simulink model "PMSM_SMO"  (Simulink 10.0)
settings: Solver=ode45  StartTime=0.0  StopTime=0.1  RelTol=1e-3  EnableMultiTasking=on
libraries: powerlib x11, simulink x1
settings Model: Creator=jzxpc  LastModifiedBy=bhisma
settings DataIOCC: LimitDataPoints=on  SignalLoggingSaveFormat=ModelDataLogs
settings OptimizationCC: ExpressionDepthLimit=2147483647  InitFltsAndDblsToZero=on
settings DebuggingCC: SaveWithParameterizedLinksMsg=none  SignalResolutionControl=TryResolveAllWithWarning  FcnCallInpInsideContextMsg=warning  StateNameClashWarn=warning
settings SFSimCC: SimParseCustomCode=off
settings GRTTargetCC: TargetFcnLib=ansi_tfl_tmw.mat  GeneratePreprocessorConditionals=Disable all
settings ConfigComp: CovExternalEMLEnable=off

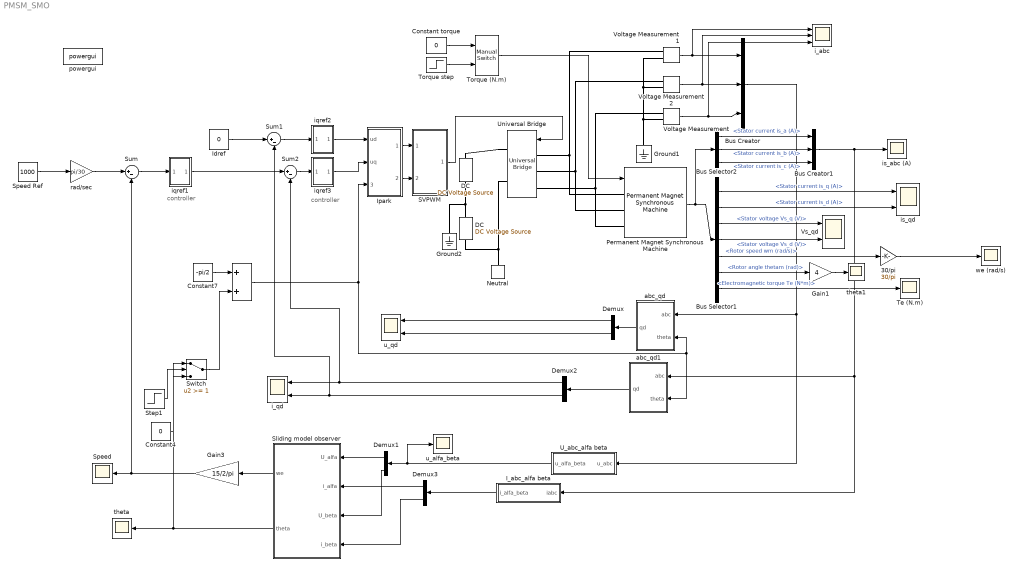
== system PMSM_SMO ==
  note: controller
  note: controller
  "  " : Sum
  30/pi : Gain  Gain=30/pi
  Bus Creator : BusCreator  Inputs=3
  Bus Creator1 : BusCreator  Inputs=3
  Bus Selector1 : BusSelector  OutputSignals=Stator current is_q (A),Stator current is_d (A),Stator voltage Vs_q (V),Stator voltage Vs_d (V),Rotor speed wm (rad/s),Rotor angle thetam (rad),Electromagnetic torque Te (N*m)
  Bus Selector2 : BusSelector  OutputSignals=Stator current is_a (A),Stator current is_b (A),Stator current is_c (A)
  Constant torque : Constant  Value=0
  Constant4 : Constant  Value=0
  Constant7 : Constant  Value=-pi/2
  DC : powerlib/Electrical Sources/DC Voltage Source  SystemSampleTime=-1  Amplitude=250  Measurements=None
      settings: SourceProductName=Simscape Electrical
  "DC " : powerlib/Electrical Sources/DC Voltage Source  SystemSampleTime=-1  Amplitude=250  Measurements=None
      settings: SourceProductName=Simscape Electrical
  Demux{,1..3} (4 alike) : Demux  Outputs=2
  Gain1 : Gain  Gain=4
  Gain3 : Gain  Gain=15/2/pi
  Ground1 : powerlib/Elements/Ground  PhysicalDomain=powersysdomain  SubClassName=unknown  LeftPortType=p1  RightPortType=p1  LConnTagsString=a
      settings: SourceProductName=Simscape Electrical
  Ground2 : powerlib/Elements/Ground  PhysicalDomain=powersysdomain  SubClassName=unknown  LeftPortType=p1  RightPortType=p1  LConnTagsString=a
      settings: SourceProductName=Simscape Electrical
  I_abc_alfa beta : Subsystem
  Idref : Constant  Value=0
  Ipark : Subsystem
  Neutral : powerlib/Elements/Neutral  PhysicalDomain=powersysdomain  SubClassName=unknown  LeftPortType=p1  RightPortType=p1  LConnTagsString=a  NodeNumber=10
      settings: SourceProductName=Simscape Electrical  SourceProductBaseCode=PS
  Permanent Magnet Synchronous Machine : powerlib/Machines/Permanent Magnet Synchronous Machine  SystemSampleTime=-1  FluxDistribution=Sinusoidal  MechanicalLoad=Torque Tm  PresetModel=No  ShowDetailedParameters=on  Resistance=1.9  Inductance=8.5e-3  dqInductances=[1e-2 1e-2]  MachineConstant=Flux linkage established by magnets (V.s)  Flux=0.353  VoltageCst=128.0542  TorqueCst=1.059  Flat=120  Mechanical=[7.24e-4 0.02e-6 2]  PolePairs=2  InitialConditions=[0,0, 0,0]  TsPowergui=0  TsBlock=-1
  SVPWM : Subsystem  TreatAsAtomicUnit=on
  Sliding model observer : Subsystem
  Speed : Scope
  Speed Ref : Constant  Value=1000
  Step1 : Step  Time=0.001  SampleTime=0
  Sum : Sum  Inputs=|+-
  Sum1 : Sum  Inputs=|+-
  Sum2 : Sum  Inputs=|+-
  Switch : Switch  Threshold=1
  Te (N.m) : Scope
  Torque (N.m) : simulink/Signal Routing/Manual Switch  SystemSampleTime=-1  sw=0  action=0  varsize=off
      settings: SourceProductName=Simulink  SourceProductBaseCode=SL
  Torque step : Step  Time=0  After=4  SampleTime=0
  U_abc_alfa beta : Subsystem
  Universal Bridge : powerlib/Power Electronics/Universal Bridge  SystemSampleTime=-1  Arms=3  SnubberResistance=1e5  SnubberCapacitance=inf  Device=IGBT / Diodes  Ron=1e-3  Lon=0  ForwardVoltages="[  0  0  ]"  ForwardVoltage=0  GTOparameters=[ 10e-6 , 20e-6 ]  IGBTparameters=[ 1e-6 , 2e-6 ]  Measurements=None  Measurements_2=None  converterType=Rectifier
      settings: SourceProductName=Simscape Electrical
  Voltage Measurement : powerlib/Measurements/Voltage Measurement  SystemSampleTime=-1  PhasorSimulation=off  OutputType=Complex  PSBequivalent=0
      settings: SourceProductName=Simscape Electrical
  Voltage Measurement1 : powerlib/Measurements/Voltage Measurement  SystemSampleTime=-1  PhasorSimulation=off  OutputType=Complex  PSBequivalent=0
      settings: SourceProductName=Simscape Electrical
  Voltage Measurement2 : powerlib/Measurements/Voltage Measurement  SystemSampleTime=-1  PhasorSimulation=off  OutputType=Complex  PSBequivalent=0
      settings: SourceProductName=Simscape Electrical
  Vs_qd : Scope  NumInputPorts=2
  abc_qd : Subsystem
  abc_qd1 : Subsystem
  i_abc : Scope  NumInputPorts=3
  "i_qd " : Scope  NumInputPorts=2
  iqref1 : Subsystem  mask(PI Controller){I=1.2, P=2, sat=[-50, 50]}
      mask prompts: I "Integral"; P "Proportional:"; sat "Minimum and maximum outputs:"
      mask init:
      | min=sat(1);max=sat(2);
      mask Display: disp('PI')
  iqref2 : Subsystem  mask(PI Controller){I=1000, P=10, sat=[-200, 200]}
      mask prompts: I "Integral"; P "Proportional:"; sat "Minimum and maximum outputs:"
      mask init:
      | min=sat(1);max=sat(2);
      mask Display: disp('PI')
  iqref3 : Subsystem  mask(PI Controller){I=1000, P=10, sat=[-200, 200]}
      mask prompts: I "Integral"; P "Proportional:"; sat "Minimum and maximum outputs:"
      mask init:
      | min=sat(1);max=sat(2);
      mask Display: disp('PI')
  is_abc (A) : Scope
  is_qd : Scope  NumInputPorts=2
  powergui : powerlib/powergui  SystemSampleTime=-1  SimulationMode=Continuous  SampleTime=50e-6  frequency=60  SPID=off  DisableSnubberDevices=off  DisableRonSwitches=off  DisableVfSwitches=off  SwTol=0  Interpol=off  frequencyindice=0  echomessages=off  HookPort=off  DisplayEquations=off  FunctionMessages=off  EnableUseOfTLC=off  x0status=blocks  RestoreLinks=warning  ResistiveCurrentMeasurement=off  Frange=[0:2:500]  Ylog=off  Xlog=on  ShowGrid=off  save=off  variable=ZData  ZoomFFT=on  StartTime=0.0  cycles=1  DisplayStyle=1  fundamental=60  FreqAxis=off  MaxFrequency=1000  frequencyindicesteady=1  RmsSteady=1  display=off  Ts=0  methode=off
      settings: SourceProductName=Simscape Electrical
  rad/sec : Gain  Gain=pi/30
  theta : Scope
  theta1 : Scope
  u_alfa_beta : Scope
  "u_qd " : Scope  NumInputPorts=2
  we (rad/s) : Scope
  wires:
  iqref2/1(Out_1) -> Ipark/1(ud)
  iqref3/1(Out_1) -> Ipark/2(uq)
  Ipark/1(ualpha) -> SVPWM/1(Ualfa)
  Ipark/2(ubeta) -> SVPWM/2(Ubeta)
  Sum/1 -> iqref1/1(In_1)
  Speed Ref/1 -> rad/sec/1
  Permanent Magnet Synchronous Machine/1 -> Bus Selector2/1, Bus Selector1/1
  Idref/1 -> Sum1/1
  Sum1/1 -> iqref2/1(In_1)
  Sum2/1 -> iqref3/1(In_1)
  iqref1/1(Out_1) -> Sum2/1
  Torque step/1 -> Torque (N.m)/2
  Constant torque/1 -> Torque (N.m)/1
  Voltage Measurement1/1 -> Bus Creator/1, i_abc/1
  Voltage Measurement2/1 -> Bus Creator/2, i_abc/2
  Voltage Measurement/1 -> Bus Creator/3, i_abc/3
  Bus Selector2/1 -> Bus Creator1/1  "<Stator current is_a (A)>"
  Bus Selector2/2 -> Bus Creator1/2  "<Stator current is_b (A)>"
  Bus Selector2/3 -> Bus Creator1/3  "<Stator current is_c (A)>"
  Bus Creator1/1 -> is_abc (A)/1, I_abc_alfa beta/1(iabc), abc_qd1/1(abc)
  Bus Selector1/1 -> is_qd/1  "<Stator current is_q (A)>"
  Bus Selector1/2 -> is_qd/2  "<Stator current is_d (A)>"
  Bus Selector1/3 -> Vs_qd/1  "<Stator voltage Vs_q (V)>"
  Bus Selector1/4 -> Vs_qd/2  "<Stator voltage Vs_d (V)>"
  Bus Selector1/5 -> 30/pi/1  "<Rotor speed wm (rad/s)>"
  Bus Selector1/6 -> Gain1/1  "<Rotor angle thetam (rad)>"
  Bus Selector1/7 -> Te (N.m)/1  "<Electromagnetic torque Te (N*m)>"
  30/pi/1 -> we (rad/s)/1
  Bus Creator/1 -> U_abc_alfa beta/1(u_abc), abc_qd/1(abc)
  Demux/1 -> "u_qd "/1
  Demux/2 -> "u_qd "/2
  abc_qd/1(qd) -> Demux/1
  Demux2/1 -> "i_qd "/1, Sum2/2
  Demux2/2 -> "i_qd "/2, Sum1/2
  abc_qd1/1(qd) -> Demux2/1
  U_abc_alfa beta/1(u_alfa_beta) -> Demux1/1, u_alfa_beta/1
  I_abc_alfa beta/1(i_alfa_beta) -> Demux3/1
  Demux1/1 -> Sliding model observer/1(U_alfa)
  Demux1/2 -> Sliding model observer/3(U_beta)
  Demux3/1 -> Sliding model observer/2(i_alfa)
  Demux3/2 -> Sliding model observer/4(i_beta)
  Gain3/1 -> Speed/1, Sum/2
  Sliding model observer/1(we) -> Gain3/1
  Sliding model observer/2(theta) -> Switch/1, theta/1
  Switch/1 -> "  "/2
  Step1/1 -> Switch/2
  Constant4/1 -> Switch/3
  Constant7/1 -> "  "/1
  "  "/1 -> Ipark/3(theta), abc_qd/2(theta), abc_qd1/2(theta)
  rad/sec/1 -> Sum/1
  SVPWM/1(Pulses) -> Universal Bridge/1
  Torque (N.m)/1 -> Permanent Magnet Synchronous Machine/1
  Gain1/1 -> theta1/1
  connections:
  Voltage Measurement1/LConn2 -- Voltage Measurement2/LConn2 -- Ground1/LConn1 -- Voltage Measurement/LConn2
  Universal Bridge/LConn1 -- Permanent Magnet Synchronous Machine/LConn1 -- Voltage Measurement1/LConn1
  Permanent Magnet Synchronous Machine/LConn2 -- Universal Bridge/LConn2 -- Voltage Measurement2/LConn1
  Universal Bridge/LConn3 -- Permanent Magnet Synchronous Machine/LConn3 -- Voltage Measurement/LConn1
  DC/RConn1 -- Ground2/LConn1 -- "DC "/LConn1
  DC/LConn1 -- Neutral/LConn1 -- Universal Bridge/RConn2
  Universal Bridge/RConn1 -- "DC "/RConn1

== system PMSM_SMO/I_abc_alfa beta ==
  iabc : Inport
  Fcn : Fcn  Expr=(2*u(1)-u(2)-u(3))/3
  Fcn1 : Fcn  Expr=(u(2)-u(3))/(3^(1/2))
  Mux2 : Mux  Inputs=2
  i_alfa_beta : Outport
  wires:
  Fcn1/1 -> Mux2/2
  Fcn/1 -> Mux2/1
  Mux2/1 -> i_alfa_beta/1
  iabc/1 -> Fcn1/1, Fcn/1

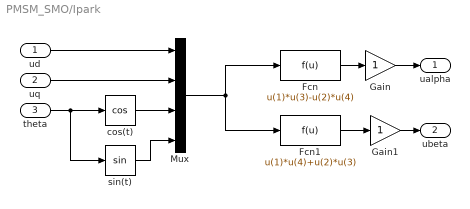
== system PMSM_SMO/Ipark ==
  ud : Inport
  uq : Inport  Port=2
  theta : Inport  Port=3
  Fcn : Fcn  Expr=u(1)*u(3)-u(2)*u(4)
  Fcn1 : Fcn  Expr=u(1)*u(4)+u(2)*u(3)
  Gain : Gain
  Gain1 : Gain
  Mux : Mux
  cos(t) : Trigonometry  Operator=cos
  sin(t) : Trigonometry
  ualpha : Outport
  ubeta : Outport  Port=2
  wires:
  ud/1 -> Mux/1
  uq/1 -> Mux/2
  cos(t)/1 -> Mux/3
  sin(t)/1 -> Mux/4
  theta/1 -> cos(t)/1, sin(t)/1
  Mux/1 -> Fcn/1, Fcn1/1
  Gain/1 -> ualpha/1
  Fcn/1 -> Gain/1
  Gain1/1 -> ubeta/1
  Fcn1/1 -> Gain1/1

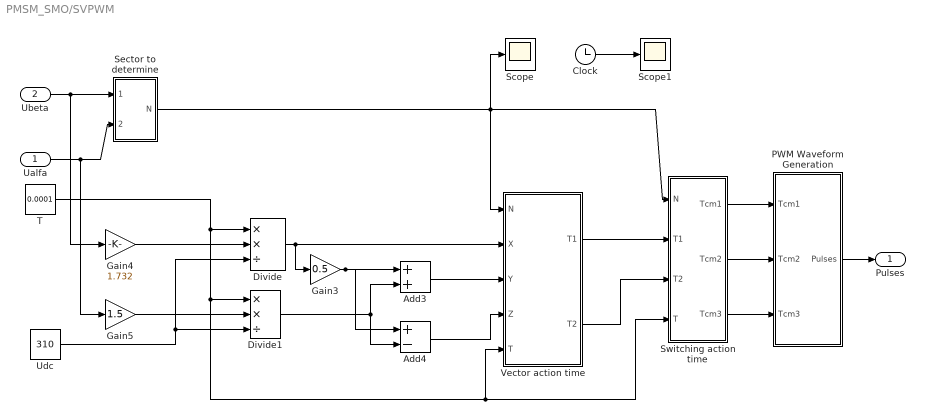
== system PMSM_SMO/SVPWM ==
  Ualfa : Inport
  Ubeta : Inport  Port=2
  Add3 : Sum
  Add4 : Sum  Inputs=+-
  Clock : Clock
  Divide : Product  Inputs=**/
  Divide1 : Product  Inputs=**/
  Gain3 : Gain  Gain=0.5
  Gain4 : Gain  Gain=1.732
  Gain5 : Gain  Gain=1.5
  PWM Waveform Generation : Subsystem
  Scope : Scope
  Scope1 : Scope
  Sector to determine : Subsystem
  Switching action time : Subsystem
  T : Constant  Value=0.0001
  Udc : Constant  Value=310
  Vector action time : Subsystem  TreatAsAtomicUnit=on
  Pulses : Outport
  wires:
  Clock/1 -> Scope1/1
  Switching action time/3(Tcm3) -> PWM Waveform Generation/3(Tcm3)
  Switching action time/2(Tcm2) -> PWM Waveform Generation/2(Tcm2)
  Switching action time/1(Tcm1) -> PWM Waveform Generation/1(Tcm1)
  Divide/1 -> Vector action time/2(X), Gain3/1
  Gain4/1 -> Divide/2
  Gain3/1 -> Add4/1, Add3/1
  Gain5/1 -> Divide1/2
  Divide1/1 -> Add4/2, Add3/2
  Add4/1 -> Vector action time/4(Z)
  Add3/1 -> Vector action time/3(Y)
  Sector to determine/1(N) -> Switching action time/1(N), Scope/1, Vector action time/1(N)
  Ubeta/1 -> Gain4/1, Sector to determine/1(Ubeta)
  Ualfa/1 -> Gain5/1, Sector to determine/2(Ualfa)
  T/1 -> Divide/1, Divide1/1, Switching action time/4(T), Vector action time/5(T)
  Udc/1 -> Divide1/3, Divide/3
  Vector action time/1(T1) -> Switching action time/2(T1)
  Vector action time/2(T2) -> Switching action time/3(T2)
  PWM Waveform Generation/1(Pulses) -> Pulses/1

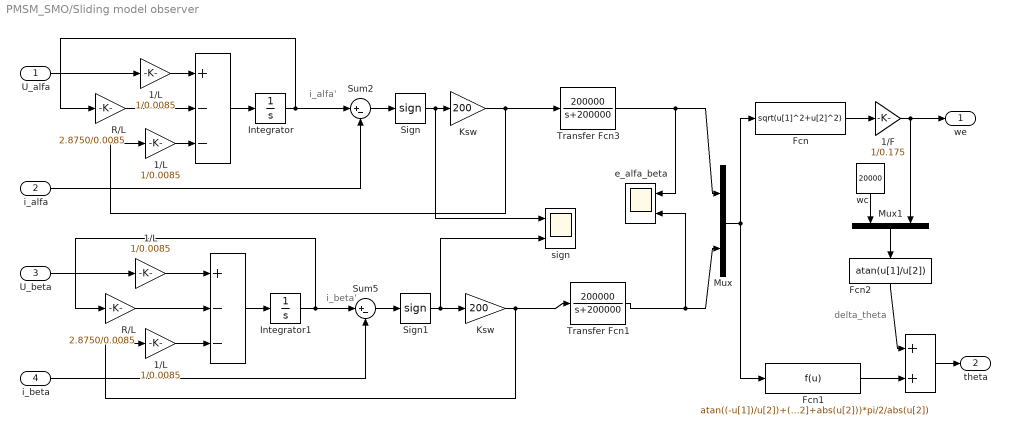
== system PMSM_SMO/Sliding model observer ==
  note: delta_theta
  note: i_beta'
  note: i_alfa'
  U_alfa : Inport
  i_alfa : Inport  Port=2
  U_beta : Inport  Port=3
  i_beta : Inport  Port=4
  " " : Sum  Inputs=+--
  "  " : Sum
  "   " : Sum  Inputs=+--
  " 1/L" : Gain  Gain=1/0.0085
  " 1/L " : Gain  Gain=1/0.0085
  1/F : Gain  Gain=1/0.175
  1/L : Gain  Gain=1/0.0085
  "1/L " : Gain  Gain=1/0.0085
  Fcn : Fcn  Expr=sqrt(u[1]^2+u[2]^2)
  Fcn1 : Fcn  Expr=atan((-u[1])/u[2])+(-u[2]+abs(u[2]))*pi/2/abs(u[2])
  Fcn2 : Fcn  Expr=atan(u[1]/u[2])
  Integrator : Integrator
  Integrator1 : Integrator
  Ksw : Gain  Gain=200
  "Ksw " : Gain  Gain=200
  Mux : Mux  Inputs=2
  Mux1 : Mux  Inputs=2
  R/L : Gain  Gain=2.8750/0.0085
  "R/L " : Gain  Gain=2.8750/0.0085
  Sign : Signum  ZeroCross=off
  Sign1 : Signum  ZeroCross=off
  Sum2 : Sum  Inputs=|+-
  Sum5 : Sum  Inputs=|+-
  Transfer Fcn1 : TransferFcn  Numerator=[200000]  Denominator=[1 200000]
  Transfer Fcn3 : TransferFcn  Numerator=[200000]  Denominator=[1 200000]
  e_alfa_beta : Scope  NumInputPorts=2
  sign : Scope  NumInputPorts=2
  wc : Constant  Value=20000
  we : Outport
  theta : Outport  Port=2
  wires:
  wc/1 -> Mux1/1
  Fcn2/1 -> "  "/1
  Mux1/1 -> Fcn2/1
  Transfer Fcn3/1 -> e_alfa_beta/1, Mux/1
  Transfer Fcn1/1 -> e_alfa_beta/2, Mux/2
  "  "/1 -> theta/1
  Fcn1/1 -> "  "/2
  Sum2/1 -> Sign/1
  1/F/1 -> we/1, Mux1/2
  " 1/L "/1 -> "   "/3
  "   "/1 -> Integrator1/1
  "R/L "/1 -> "   "/2
  " 1/L"/1 -> "   "/1
  U_beta/1 -> " 1/L"/1
  " "/1 -> Integrator/1
  "1/L "/1 -> " "/3
  R/L/1 -> " "/2
  1/L/1 -> " "/1
  U_alfa/1 -> 1/L/1
  Fcn/1 -> 1/F/1
  Mux/1 -> Fcn1/1, Fcn/1
  i_beta/1 -> Sum5/2
  i_alfa/1 -> Sum2/2
  "Ksw "/1 -> Transfer Fcn1/1, " 1/L "/1
  Sign1/1 -> sign/2, "Ksw "/1
  Sum5/1 -> Sign1/1
  Integrator1/1 -> "R/L "/1, Sum5/1
  Ksw/1 -> Transfer Fcn3/1, "1/L "/1
  Sign/1 -> sign/1, Ksw/1
  Integrator/1 -> R/L/1, Sum2/1

== system PMSM_SMO/U_abc_alfa beta ==
  u_abc : Inport
  Fcn : Fcn  Expr=(2*u(1)-u(2)-u(3))/3
  Fcn1 : Fcn  Expr=(u(2)-u(3))/(3^(1/2))
  Mux2 : Mux  Inputs=2
  u_alfa_beta : Outport
  wires:
  Fcn1/1 -> Mux2/2
  Fcn/1 -> Mux2/1
  Mux2/1 -> u_alfa_beta/1
  u_abc/1 -> Fcn1/1, Fcn/1

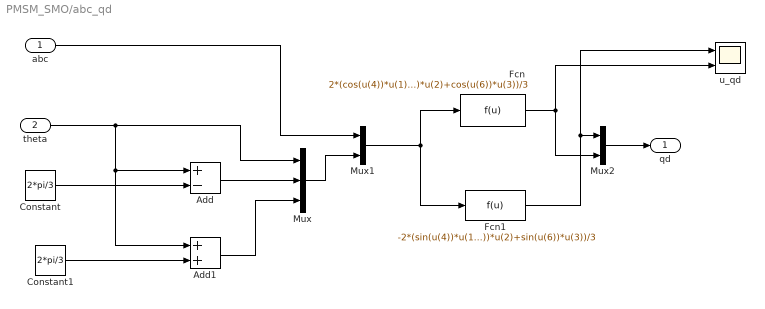
== system PMSM_SMO/abc_qd ==
  abc : Inport
  theta : Inport  Port=2
  Add : Sum  Inputs=+-
  Add1 : Sum
  Constant : Constant  Value=2*pi/3
  Constant1 : Constant  Value=2*pi/3
  Fcn : Fcn  Expr=2*(cos(u(4))*u(1)+cos(u(5))*u(2)+cos(u(6))*u(3))/3
  Fcn1 : Fcn  Expr=-2*(sin(u(4))*u(1)+sin(u(5))*u(2)+sin(u(6))*u(3))/3
  Mux : Mux  Inputs=3
  Mux1 : Mux  Inputs=2
  Mux2 : Mux  Inputs=2
  "u_qd " : Scope  NumInputPorts=2
  qd : Outport
  wires:
  Fcn1/1 -> "u_qd "/1, Mux2/1
  Fcn/1 -> "u_qd "/2, Mux2/2
  Mux2/1 -> qd/1
  Mux1/1 -> Fcn1/1, Fcn/1
  abc/1 -> Mux1/1
  Mux/1 -> Mux1/2
  Add1/1 -> Mux/3
  Add/1 -> Mux/2
  theta/1 -> Add/1, Add1/1, Mux/1
  Constant/1 -> Add/2
  Constant1/1 -> Add1/2

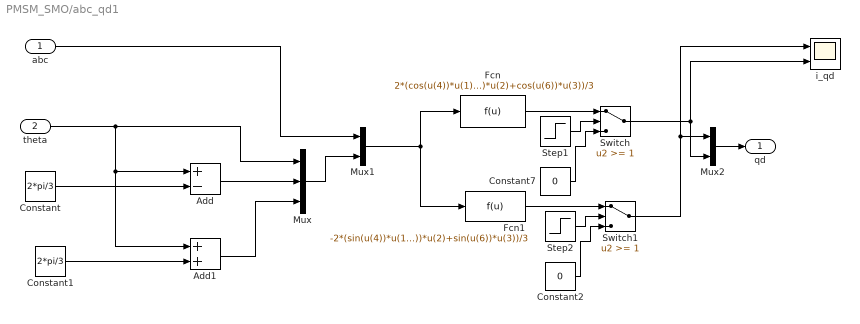
== system PMSM_SMO/abc_qd1 ==
  abc : Inport
  theta : Inport  Port=2
  Add : Sum  Inputs=+-
  Add1 : Sum
  Constant : Constant  Value=2*pi/3
  Constant1 : Constant  Value=2*pi/3
  Constant2 : Constant  Value=0
  Constant7 : Constant  Value=0
  Fcn : Fcn  Expr=2*(cos(u(4))*u(1)+cos(u(5))*u(2)+cos(u(6))*u(3))/3
  Fcn1 : Fcn  Expr=-2*(sin(u(4))*u(1)+sin(u(5))*u(2)+sin(u(6))*u(3))/3
  Mux : Mux  Inputs=3
  Mux1 : Mux  Inputs=2
  Mux2 : Mux  Inputs=2
  Step1 : Step  Time=0.0001  SampleTime=0
  Step2 : Step  Time=0.0001  SampleTime=0
  Switch : Switch  Threshold=1
  Switch1 : Switch  Threshold=1
  "i_qd " : Scope  NumInputPorts=2
  qd : Outport
  wires:
  Switch1/1 -> "i_qd "/1, Mux2/1
  Constant2/1 -> Switch1/3
  Step2/1 -> Switch1/2
  Fcn1/1 -> Switch1/1
  Constant7/1 -> Switch/3
  Step1/1 -> Switch/2
  Switch/1 -> "i_qd "/2, Mux2/2
  Fcn/1 -> Switch/1
  Mux2/1 -> qd/1
  Mux1/1 -> Fcn1/1, Fcn/1
  abc/1 -> Mux1/1
  Mux/1 -> Mux1/2
  Add1/1 -> Mux/3
  Add/1 -> Mux/2
  theta/1 -> Add/1, Add1/1, Mux/1
  Constant/1 -> Add/2
  Constant1/1 -> Add1/2

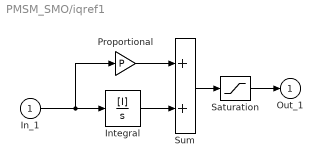
== system PMSM_SMO/iqref1 ==
  In_1 : Inport
  Integral : TransferFcn  Numerator=[I]  Denominator=[1 0]
  Proportional : Gain  Gain=P  SaturateOnIntegerOverflow=on  OutDataTypeStr=Inherit: Same as input  ParamDataTypeStr=Inherit: Same as input
  Saturation : Saturate  UpperLimit=max  LowerLimit=min
  Sum : Sum  SaturateOnIntegerOverflow=on  InputSameDT=on  OutDataTypeStr=Inherit: Same as first input
  Out_1 : Outport  InitialOutput=0
  wires:
  Saturation/1 -> Out_1/1
  Sum/1 -> Saturation/1
  Proportional/1 -> Sum/1
  In_1/1 -> Proportional/1, Integral/1
  Integral/1 -> Sum/2

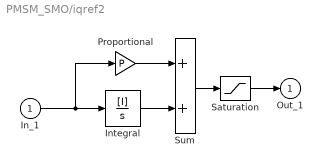
== system PMSM_SMO/iqref2 ==
  In_1 : Inport
  Integral : TransferFcn  Numerator=[I]  Denominator=[1 0]
  Proportional : Gain  Gain=P  SaturateOnIntegerOverflow=on  OutDataTypeStr=Inherit: Same as input  ParamDataTypeStr=Inherit: Same as input
  Saturation : Saturate  UpperLimit=max  LowerLimit=min
  Sum : Sum  SaturateOnIntegerOverflow=on  InputSameDT=on  OutDataTypeStr=Inherit: Same as first input
  Out_1 : Outport  InitialOutput=0
  wires:
  Saturation/1 -> Out_1/1
  Sum/1 -> Saturation/1
  Proportional/1 -> Sum/1
  In_1/1 -> Proportional/1, Integral/1
  Integral/1 -> Sum/2

== system PMSM_SMO/iqref3 ==
  In_1 : Inport
  Integral : TransferFcn  Numerator=[I]  Denominator=[1 0]
  Proportional : Gain  Gain=P  SaturateOnIntegerOverflow=on  OutDataTypeStr=Inherit: Same as input  ParamDataTypeStr=Inherit: Same as input
  Saturation : Saturate  UpperLimit=max  LowerLimit=min
  Sum : Sum  SaturateOnIntegerOverflow=on  InputSameDT=on  OutDataTypeStr=Inherit: Same as first input
  Out_1 : Outport  InitialOutput=0
  wires:
  Saturation/1 -> Out_1/1
  Sum/1 -> Saturation/1
  Proportional/1 -> Sum/1
  In_1/1 -> Proportional/1, Integral/1
  Integral/1 -> Sum/2

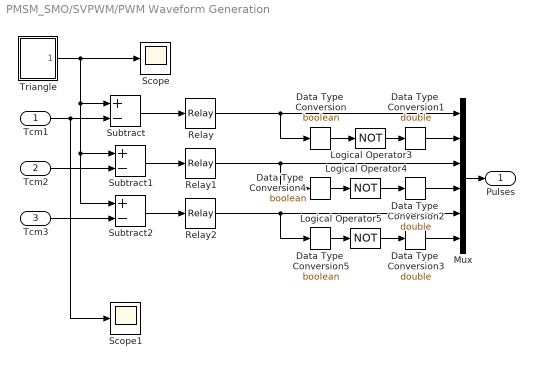
== system PMSM_SMO/SVPWM/PWM Waveform Generation ==
  Tcm1 : Inport
  Tcm2 : Inport  Port=2
  Tcm3 : Inport  Port=3
  Data Type  Conversion : DataTypeConversion  OutDataTypeStr=boolean  SaturateOnIntegerOverflow=on  RndMeth=Zero
  Data Type  Conversion1 : DataTypeConversion  OutDataTypeStr=double  SaturateOnIntegerOverflow=on  RndMeth=Zero
  Data Type  Conversion2 : DataTypeConversion  OutDataTypeStr=double  SaturateOnIntegerOverflow=on  RndMeth=Zero
  Data Type  Conversion3 : DataTypeConversion  OutDataTypeStr=double  SaturateOnIntegerOverflow=on  RndMeth=Zero
  Data Type  Conversion4 : DataTypeConversion  OutDataTypeStr=boolean  SaturateOnIntegerOverflow=on  RndMeth=Zero
  Data Type  Conversion5 : DataTypeConversion  OutDataTypeStr=boolean  SaturateOnIntegerOverflow=on  RndMeth=Zero
  Logical Operator3 : Logic  Operator=NOT
  Logical Operator4 : Logic  Operator=NOT
  Logical Operator5 : Logic  Operator=NOT
  Mux : Mux  Inputs=6
  Relay : Relay
  Relay1 : Relay
  Relay2 : Relay
  Scope : Scope
  Scope1 : Scope
  Subtract : Sum  Inputs=+-
  Subtract1 : Sum  Inputs=+-
  Subtract2 : Sum  Inputs=+-
  Triangle : Subsystem
  Pulses : Outport  InitialOutput=0
  wires:
  Tcm3/1 -> Subtract2/2
  Tcm2/1 -> Subtract1/2
  Tcm1/1 -> Subtract/2, Scope1/1
  Triangle/1(wave) -> Subtract1/1, Subtract2/1, Subtract/1, Scope/1
  Subtract2/1 -> Relay2/1
  Subtract1/1 -> Relay1/1
  Subtract/1 -> Relay/1
  Mux/1 -> Pulses/1
  Relay/1 -> Mux/1, Data Type  Conversion/1
  Relay1/1 -> Mux/3, Data Type  Conversion4/1
  Relay2/1 -> Mux/5, Data Type  Conversion5/1
  Data Type  Conversion/1 -> Logical Operator3/1
  Logical Operator3/1 -> Data Type  Conversion1/1
  Data Type  Conversion1/1 -> Mux/2
  Logical Operator4/1 -> Data Type  Conversion2/1
  Data Type  Conversion2/1 -> Mux/4
  Logical Operator5/1 -> Data Type  Conversion3/1
  Data Type  Conversion3/1 -> Mux/6
  Data Type  Conversion4/1 -> Logical Operator4/1
  Data Type  Conversion5/1 -> Logical Operator5/1

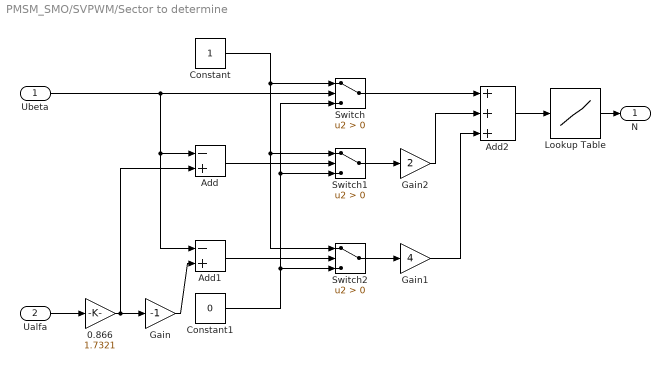
== system PMSM_SMO/SVPWM/Sector to determine ==
  Ubeta : Inport
  Ualfa : Inport  Port=2
  0.866 : Gain  Gain=1.7321
  Add : Sum  Inputs=-+
  Add1 : Sum  Inputs=-+
  Add2 : Sum  Inputs=+++
  Constant : Constant
  Constant1 : Constant  Value=0
  Gain : Gain  Gain=-1
  Gain1 : Gain  Gain=4
  Gain2 : Gain  Gain=2
  Lookup Table : Lookup  InputValues=[1 2 3 4 5 6]  Table=[3 1 5 4 6 2]
  Switch : Switch  Criteria=u2 > Threshold
  Switch1 : Switch  Criteria=u2 > Threshold
  Switch2 : Switch  Criteria=u2 > Threshold
  N : Outport
  wires:
  Ualfa/1 -> 0.866/1
  Ubeta/1 -> Switch/2, Add1/1, Add/1
  Switch/1 -> Add2/1
  Gain2/1 -> Add2/2
  Gain1/1 -> Add2/3
  Switch1/1 -> Gain2/1
  Switch2/1 -> Gain1/1
  Gain/1 -> Add1/2
  0.866/1 -> Gain/1, Add/2
  Add1/1 -> Switch2/2
  Add/1 -> Switch1/2
  Constant1/1 -> Switch2/3, Switch1/3, Switch/3
  Constant/1 -> Switch1/1, Switch2/1, Switch/1
  Lookup Table/1 -> N/1
  Add2/1 -> Lookup Table/1

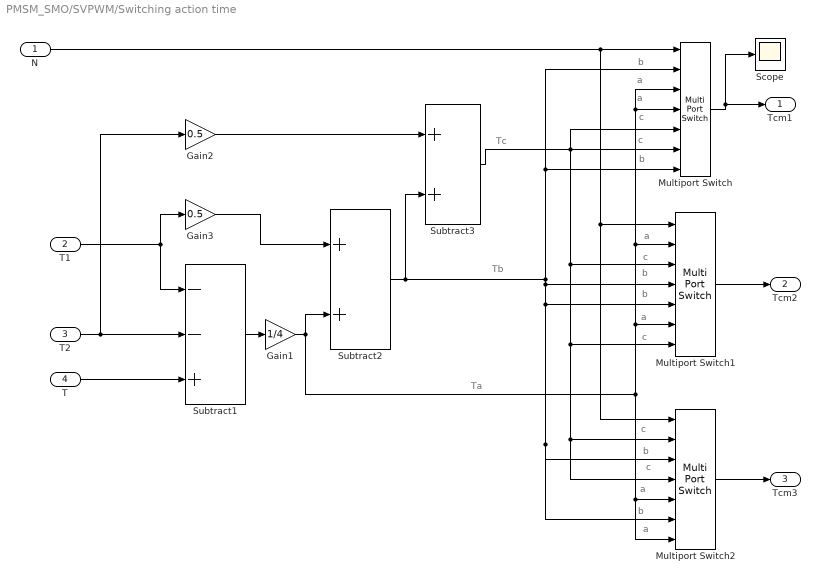
== system PMSM_SMO/SVPWM/Switching action time ==
  note: a
  note: b
  note: a
  note: c
  note: b
  note: c
  note: c
  note: a
  note: b
  note: b
  note: c
  note: a
  note: b
  note: c
  note: c
  note: a
  note: a
  note: b
  note: Tc
  note: Tb
  note: Ta
  N : Inport
  T1 : Inport  Port=2
  T2 : Inport  Port=3
  T : Inport  Port=4
  Gain1 : Gain  Gain=1/4
  Gain2 : Gain  Gain=0.5
  Gain3 : Gain  Gain=0.5
  Multiport Switch : MultiPortSwitch  Inputs=6
  Multiport Switch1 : MultiPortSwitch  Inputs=6
  Multiport Switch2 : MultiPortSwitch  Inputs=6
  Scope : Scope
  Subtract1 : Sum  Inputs=--+
  Subtract2 : Sum
  Subtract3 : Sum
  Tcm1 : Outport
  Tcm2 : Outport  Port=2
  Tcm3 : Outport  Port=3
  wires:
  Subtract3/1 -> Multiport Switch2/4, Multiport Switch2/2, Multiport Switch1/7, Multiport Switch1/3, Multiport Switch/6, Multiport Switch/5
  Gain1/1 -> Multiport Switch/4, Multiport Switch/3, Multiport Switch1/2, Multiport Switch1/6, Multiport Switch2/7, Multiport Switch2/5, Subtract2/2
  Gain2/1 -> Subtract3/1
  Multiport Switch2/1 -> Tcm3/1
  Multiport Switch1/1 -> Tcm2/1
  Multiport Switch/1 -> Scope/1, Tcm1/1
  N/1 -> Multiport Switch1/1, Multiport Switch2/1, Multiport Switch/1
  Subtract2/1 -> Multiport Switch2/3, Multiport Switch2/6, Multiport Switch1/5, Multiport Switch1/4, Multiport Switch/7, Multiport Switch/2, Subtract3/2
  Subtract1/1 -> Gain1/1
  Gain3/1 -> Subtract2/1
  T1/1 -> Subtract1/1, Gain3/1
  T/1 -> Subtract1/3
  T2/1 -> Subtract1/2, Gain2/1

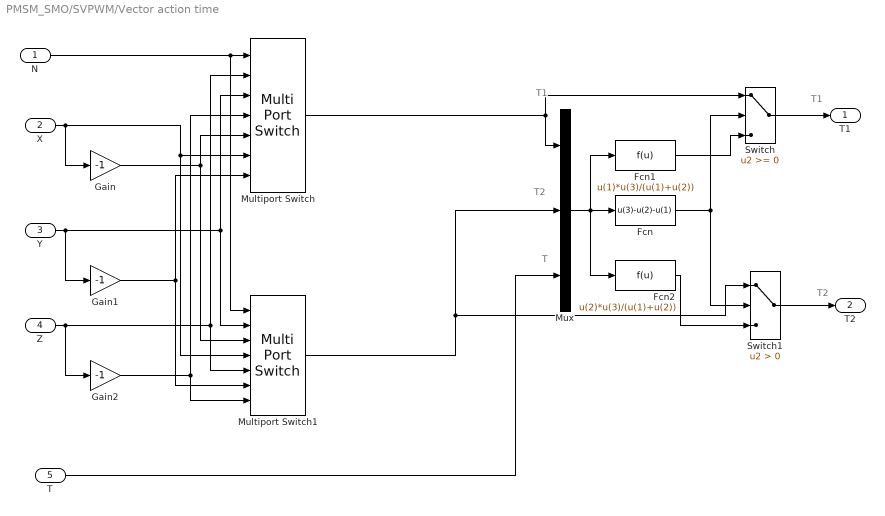
== system PMSM_SMO/SVPWM/Vector action time ==
  note: T1
  note: T2
  note: T
  note: T1
  note: T2
  N : Inport
  X : Inport  Port=2
  Y : Inport  Port=3
  Z : Inport  Port=4
  T : Inport  Port=5
  Fcn : Fcn  Expr=u(3)-u(2)-u(1)
  Fcn1 : Fcn  Expr=u(1)*u(3)/(u(1)+u(2))
  Fcn2 : Fcn  Expr=u(2)*u(3)/(u(1)+u(2))
  Gain : Gain  Gain=-1
  Gain1 : Gain  Gain=-1
  Gain2 : Gain  Gain=-1
  Multiport Switch : MultiPortSwitch  Inputs=6
  Multiport Switch1 : MultiPortSwitch  Inputs=6
  Mux : Mux  Inputs=3
  Switch : Switch
  Switch1 : Switch  Criteria=u2 > Threshold
  T1 : Outport
  T2 : Outport  Port=2
  wires:
  Gain1/1 -> Multiport Switch/7, Multiport Switch1/6
  Gain2/1 -> Multiport Switch1/7, Multiport Switch/4
  Gain/1 -> Multiport Switch/5, Multiport Switch1/3
  X/1 -> Multiport Switch/6, Multiport Switch1/4, Gain/1
  Z/1 -> Multiport Switch1/5, Multiport Switch/2, Gain2/1
  Y/1 -> Multiport Switch/3, Multiport Switch1/2, Gain1/1
  N/1 -> Multiport Switch1/1, Multiport Switch/1
  Multiport Switch1/1 -> Switch1/1, Mux/2
  Multiport Switch/1 -> Mux/1, Switch/1
  T/1 -> Mux/3
  Mux/1 -> Fcn/1, Fcn1/1, Fcn2/1
  Fcn/1 -> Switch/2, Switch1/2
  Fcn1/1 -> Switch/3
  Fcn2/1 -> Switch1/3
  Switch/1 -> T1/1
  Switch1/1 -> T2/1

== system PMSM_SMO/SVPWM/PWM Waveform Generation/Triangle ==
  Integrator : Integrator
  Pulse Generator : DiscretePulseGenerator  PulseType=Time based  Period=0.0002  PulseWidth=50
  Pulse Generator1 : DiscretePulseGenerator  PulseType=Time based  Period=0.0002  PulseWidth=50  PhaseDelay=0.0001
  Sum1 : Sum  Inputs=|+-  SaturateOnIntegerOverflow=on
  wave : Outport
  wires:
  Pulse Generator/1 -> Sum1/1
  Pulse Generator1/1 -> Sum1/2
  Sum1/1 -> Integrator/1
  Integrator/1 -> wave/1
